simulink model "P4"  (R2024a)
settings: Solver=ode45  StartTime=0.0  StopTime=5  RelTol=1e-3
settings Model: Creator=ahmad  LastModifiedBy=ahmad

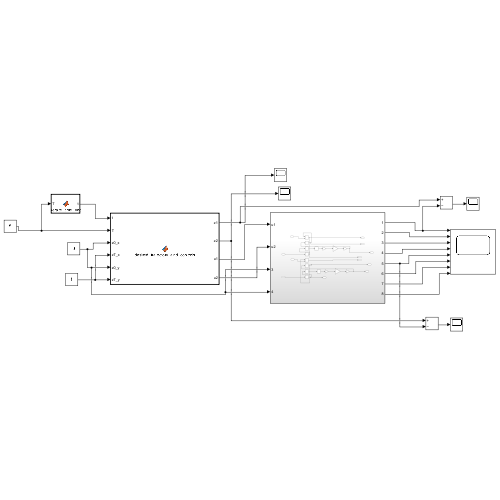
[thumbnail: Simulink's stored preview of the top-level diagram]
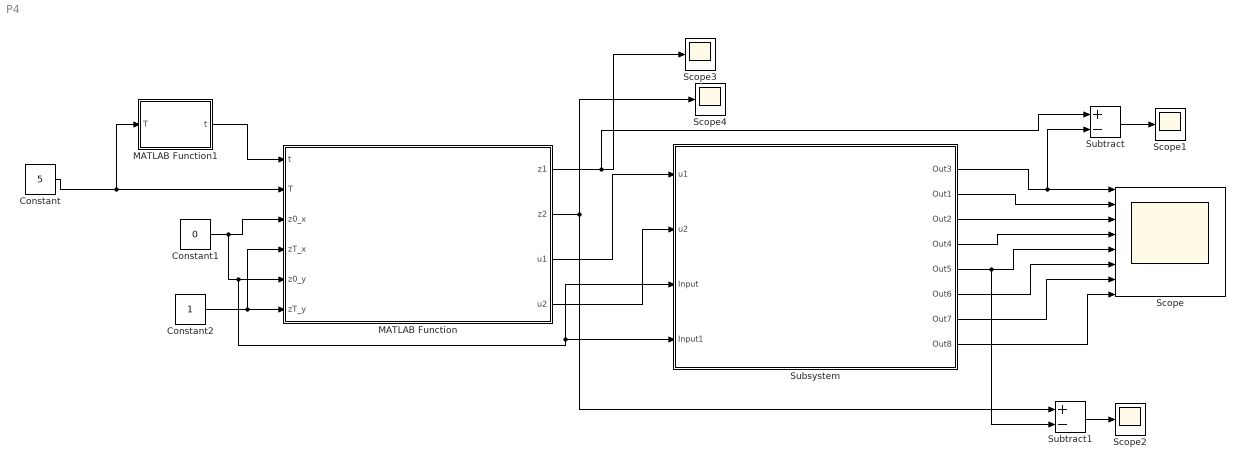
== system P4 ==
  Constant : Constant  Value=5
  Constant1 : Constant  Value=0
  Constant2 : Constant
  MATLAB Function : MATLAB Function  TreatAsAtomicUnit=on
  MATLAB Function1 : MATLAB Function  TreatAsAtomicUnit=on
  Scope : Scope  NumInputPorts=8
  Scope{1..4} (4 alike) : Scope
  Subsystem : Subsystem
  Subtract : Sum  Inputs=+-
  Subtract1 : Sum  Inputs=+-
  wires:
  MATLAB Function/3(u1) -> Subsystem/1(u1)
  MATLAB Function/4(u2) -> Subsystem/2(u2)
  Constant/1 -> MATLAB Function/2(T), MATLAB Function1/1(T)
  Constant1/1 -> Subsystem/4(Input1), Subsystem/3(Input), MATLAB Function/5(z0_y), MATLAB Function/3(z0_x)
  Constant2/1 -> MATLAB Function/4(zT_x), MATLAB Function/6(zT_y)
  MATLAB Function1/1(t) -> MATLAB Function/1(t)
  MATLAB Function/1(z1) -> Scope3/1, Subtract/1
  MATLAB Function/2(z2) -> Scope4/1, Subtract1/1
  Subsystem/1(Out3) -> Subtract/2, Scope/1
  Subsystem/2(Out1) -> Scope/2
  Subsystem/3(Out2) -> Scope/3
  Subsystem/4(Out4) -> Scope/4
  Subsystem/5(Out5) -> Subtract1/2, Scope/5
  Subsystem/6(Out6) -> Scope/6
  Subsystem/7(Out7) -> Scope/7
  Subsystem/8(Out8) -> Scope/8
  Subtract/1 -> Scope1/1
  Subtract1/1 -> Scope2/1

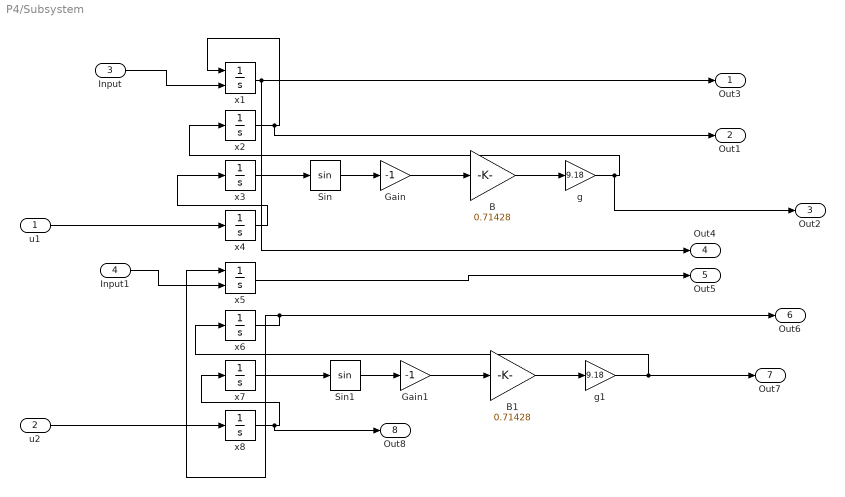
== system P4/Subsystem ==
  u1 : Inport
  u2 : Inport  Port=2
  Input : Inport  Port=3
  Input1 : Inport  Port=4
  B : Gain  Gain=0.71428
  B1 : Gain  Gain=0.71428
  Gain : Gain  Gain=-1
  Gain1 : Gain  Gain=-1
  Sin : Trigonometry
  Sin1 : Trigonometry
  g : Gain  Gain=9.18
  g1 : Gain  Gain=9.18
  x1 : Integrator  InitialConditionSource=external
  x{2..4,6..8} (6 alike) : Integrator
  x5 : Integrator  InitialConditionSource=external
  Out3 : Outport
  Out1 : Outport  Port=2
  Out2 : Outport  Port=3
  Out4 : Outport  Port=4
  Out5 : Outport  Port=5
  Out6 : Outport  Port=6
  Out7 : Outport  Port=7
  Out8 : Outport  Port=8
  wires:
  x2/1 -> Out1/1, x1/1
  B1/1 -> g1/1
  Gain1/1 -> B1/1
  x6/1 -> x5/1, Out6/1
  g/1 -> Out2/1, x2/1
  Sin1/1 -> Gain1/1
  B/1 -> g/1
  x8/1 -> Out8/1, x7/1
  x4/1 -> x3/1
  x3/1 -> Sin/1
  Gain/1 -> B/1
  x7/1 -> Sin1/1
  g1/1 -> x6/1, Out7/1
  x5/1 -> Out5/1
  Sin/1 -> Gain/1
  x1/1 -> Out4/1, Out3/1
  u2/1 -> x8/1
  u1/1 -> x4/1
  Input/1 -> x1/2
  Input1/1 -> x5/2

== matlab function P4/MATLAB Function1 ==
  data: T input; t output
function t = generate_time_vector(T)
    % Inputs: T is the total time
    % Outputs: t is a time vector
    t = linspace(0, T, 100);
end

== matlab function P4/MATLAB Function ==
  data: t input; z1 output; T input; z0_x input; zT_x input; z2 output; z0_y input; zT_y input; u1 output; u2 output
function [z1, z2, u1, u2] = desired_trajectory_and_controls(t, T, z0_x, zT_x, z0_y, zT_y)
% DESIRED_TRAJECTORY_AND_CONTROLS Computes the desired trajectories and controls
% for the ball-on-plate system for both x- and y-directions.
%
% Inputs:
%   t     - Time variable (scalar or vector)
%   T     - Transition time
%   z0_x  - Initial position in x-direction
%   zT_x  - Target position in x-direction
%   z0_y  - Initial position in y-direction
%   zT_y  - Target position in y-direction
%
% Outputs:
%   z1    - Desired trajectory for x-direction
%   z2    - Desired trajectory for y-direction
%   u1    - Control input for x-direction (fourth derivative of z1)
%   u2    - Control input for y-direction (fourth derivative of z2)

    % Coefficients for the polynomial trajectory
    p5 = 126;
    p6 = -420;
    p7 = 540;
    p8 = -315;
    p9 = 70;

    % Normalized time (t/T)
    tau = t / T;

    % Desired trajectory in x-direction (z1)
    z1 = z0_x + (zT_x - z0_x) * (p5 * tau.^5 + p6 * tau.^6 + p7 * tau.^7 + p8 * tau.^8 + p9 * tau.^9);
    % Desired trajectory in y-direction (z2)
    z2 = z0_y + (zT_y - z0_y) * (p5 * tau.^5 + p6 * tau.^6 + p7 * tau.^7 + p8 * tau.^8 + p9 * tau.^9);

    % Control input in x-direction (u1)
    u1 = (zT_x - z0_x) / T^4 * ( ...
        120 * p5 * tau + ...
        360 * p6 * tau.^2 + ...
        840 * p7 * tau.^3 + ...
        1680 * p8 * tau.^4 + ...
        3024 * p9 * tau.^5 ...
    );

    % Control input in y-direction (u2)
    u2 = (zT_y - z0_y) / T^4 * ( ...
        120 * p5 * tau + ...
        360 * p6 * tau.^2 + ...
        840 * p7 * tau.^3 + ...
        1680 * p8 * tau.^4 + ...
        3024 * p9 * tau.^5 ...
    );

end
